simulink model "Sistema"  (R2020a)
settings: Solver=VariableStepAuto  StartTime=0.0  StopTime=100  RelTol=1e-3
libraries: simulink x1
settings Model: Creator=leidy  LastModifiedBy=leidy

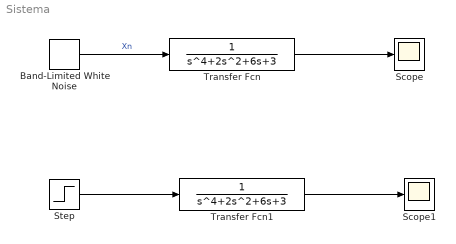
== system Sistema ==
  Band-Limited White Noise : simulink/Sources/Band-Limited White Noise  Cov=[20]  Ts=10  seed=[23341]
  Scope : Scope
  Scope1 : Scope
  Step : Step  SampleTime=0.1
  Transfer Fcn : TransferFcn  Denominator=[1 0 2 6 3]
  Transfer Fcn1 : TransferFcn  Denominator=[1 0 2 6 3]
  wires:
  Transfer Fcn/1 -> Scope/1
  Band-Limited White Noise/1 -> Transfer Fcn/1  "Xn"
  Transfer Fcn1/1 -> Scope1/1
  Step/1 -> Transfer Fcn1/1
